simulink model "system_model"  (R2024b)
settings: Solver=VariableStepAuto  StartTime=0.0  StopTime=50  RelTol=1e-3
values from neighbouring files (symbols this model uses):
  a = -21212/c    (= -13.249219238)    [Controller.m]    (also in Controller2.m; Controller_motor_only.m = -15.4812967581; motor_control.m)
  b = 21104/c    (= 13.1817613991)    [Controller.m]    (also in Controller2.m; Controller_motor_only.m = 15.421446384; motor_control.m)
  d = -1599/c    (= -0.998750780762)    [Controller.m]    (also in Controller2.m; Controller_motor_only.m = 0.995012468828; motor_control.m)
  K = -F(1:2)    [State_Space_Controller.m]
  N = -F(3)    [State_Space_Controller.m]
  Ts = 0.01    [Controller.m]    (also in Controller2.m; Controller_motor_only.m; State_Space_Controller.m; dist_translate.m)
undefined symbols (not defined in the file or in its folder): dspblkCoreblockFVToolHelper, gcbh
libraries: cstblocks x2
settings Model: Creator=alexb  LastModifiedBy=ethan

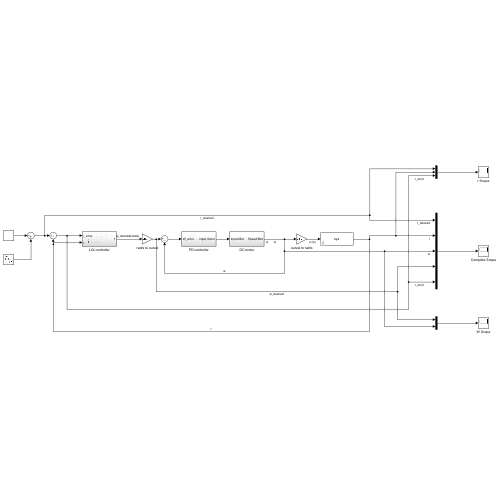
[thumbnail: Simulink's stored preview of the top-level diagram]
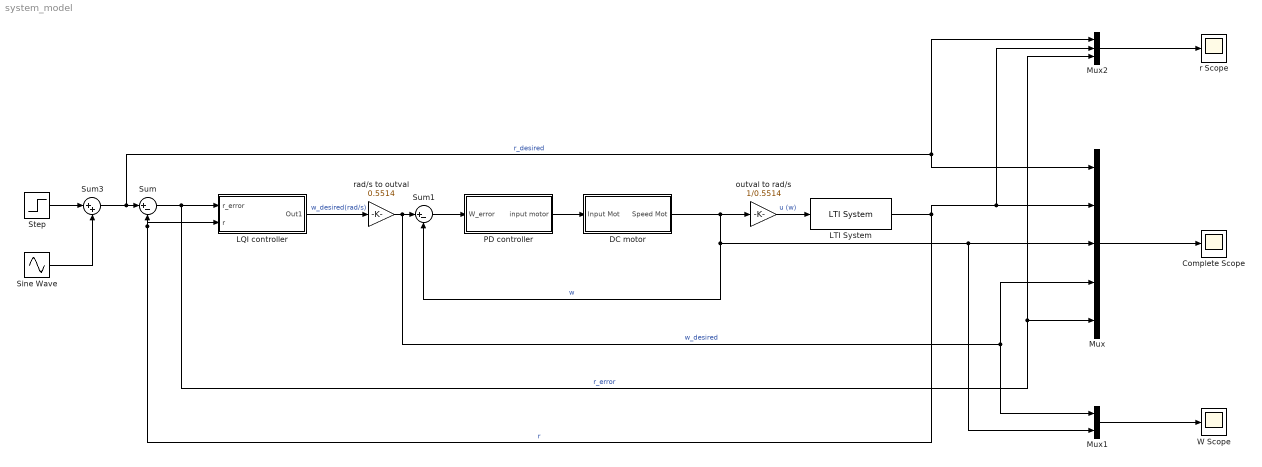
== system system_model ==
  Complete Scope : Scope
  DC motor : Subsystem
  LQI controller : Subsystem
  LTI System : cstblocks/LTI System  sys=sys  IC=[]  PadeOrder=0
  Mux : Mux  Inputs=5
  Mux1 : Mux  Inputs=2
  Mux2 : Mux  Inputs=3
  PD controller : Subsystem
  Sine Wave : Sin  Amplitude=0  Frequency=0.5  SampleTime=0
  Step : Step  Time=20  Before=0.1  After=0.13  SampleTime=0
  Sum : Sum  Inputs=|+-
  Sum1 : Sum  Inputs=|+-
  Sum3 : Sum  Inputs=|++
  W Scope : Scope
  outval to rad/s : Gain  Gain=1/0.5514
  r Scope : Scope
  rad/s to outval : Gain  Gain=0.5514
  wires:
  Sum1/1 -> PD controller/1(W_error)
  PD controller/1(input motor) -> DC motor/1(Input Mot)
  DC motor/1(Speed Mot) -> outval to rad/s/1, Mux/3, Mux1/2, Sum1/2  "w"
  Mux/1 -> Complete Scope/1
  Sum/1 -> Mux/5, Mux2/3, LQI controller/1(r_error)  "r_error"
  Step/1 -> Sum3/1
  LTI System/1 -> Mux2/2, Mux/2, Sum/2, LQI controller/2(r)  "r"
  LQI controller/1(Out1) -> rad/s to outval/1  "w_desired(rad/s)"
  Mux1/1 -> W Scope/1
  Mux2/1 -> r Scope/1
  Sum3/1 -> Mux/1, Mux2/1, Sum/1  "r_desired"
  Sine Wave/1 -> Sum3/2
  outval to rad/s/1 -> LTI System/1  "u (w)"
  rad/s to outval/1 -> Mux/4, Mux1/1, Sum1/1  "w_desired"

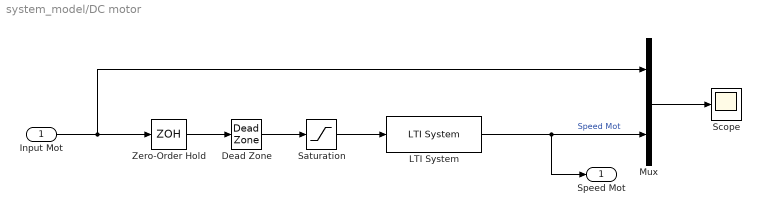
== system system_model/DC motor ==
  Input Mot : Inport
  Dead Zone : DeadZone  LowerValue=-1.75  UpperValue=1.7
  LTI System : cstblocks/LTI System  sys=Mc  IC=[]  PadeOrder=0
  Mux : Mux  Inputs=2
  Saturation : Saturate  UpperLimit=8.30  LowerLimit=-8.42
  Scope : Scope
  Zero-Order Hold : ZeroOrderHold  SampleTime=0.01
  Speed Mot : Outport
  wires:
  Input Mot/1 -> Mux/1, Zero-Order Hold/1
  Mux/1 -> Scope/1
  LTI System/1 -> Speed Mot/1, Mux/2  "Speed Mot"
  Dead Zone/1 -> Saturation/1
  Zero-Order Hold/1 -> Dead Zone/1
  Saturation/1 -> LTI System/1

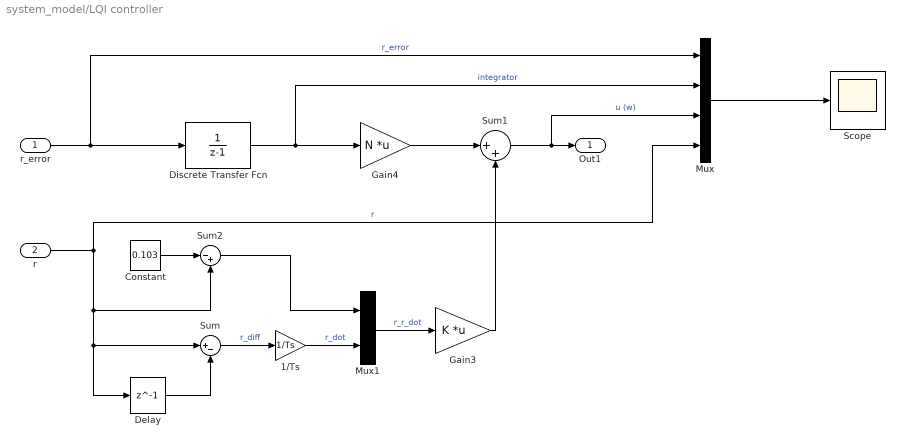
== system system_model/LQI controller ==
  r_error : Inport
  r : Inport  Port=2
  1/Ts : Gain  Gain=1/Ts
  Constant : Constant  Value=0.103
  Delay : Delay  DelayLength=1  InputProcessing=Columns as channels (frame based)
  Discrete Transfer Fcn : DiscreteTransferFcn  LoadFcn=dspblkCoreblockFVToolHelper(gcbh,'load');  Denominator=[1 -1]
      settings: CopyFcn=dspblkCoreblockFVToolHelper(gcbh,'copy');  DeleteFcn=dspblkCoreblockFVToolHelper(gcbh,'close');  ModelCloseFcn=dspblkCoreblockFVToolHelper(gcbh,'close');  PreSaveFcn=dspblkCoreblockFVToolHelper(gcbh,'presave');  PostSaveFcn=dspblkCoreblockFVToolHelper(gcbh,'postsave');  CloseFcn=dspblkCoreblockFVToolHelper(gcbh,'close');
  Gain3 : Gain  Gain=K  Multiplication=Matrix(K*u)
  Gain4 : Gain  Gain=N  Multiplication=Matrix(K*u)
  Mux : Mux
  Mux1 : Mux  Inputs=2
  Scope : Scope
  Sum : Sum  Inputs=|+-
  Sum1 : Sum  Inputs=|++
  Sum2 : Sum  Inputs=|-+
  Out1 : Outport
  wires:
  Mux/1 -> Scope/1
  Discrete Transfer Fcn/1 -> Mux/2, Gain4/1  "integrator"
  Gain3/1 -> Sum1/2
  Sum1/1 -> Out1/1, Mux/3  "u (w)"
  r_error/1 -> Discrete Transfer Fcn/1, Mux/1  "r_error"
  Gain4/1 -> Sum1/1
  r/1 -> Delay/1, Sum/1, Sum2/2, Mux/4  "r"
  Delay/1 -> Sum/2
  Mux1/1 -> Gain3/1  "r_r_dot"
  Sum/1 -> 1/Ts/1  "r_diff"
  1/Ts/1 -> Mux1/2  "r_dot"
  Sum2/1 -> Mux1/1
  Constant/1 -> Sum2/1

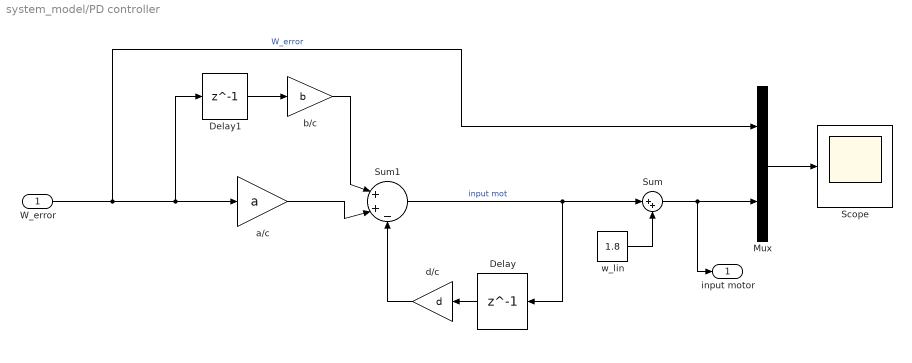
== system system_model/PD controller ==
  W_error : Inport
  Delay : Delay  DelayLength=1  InputProcessing=Columns as channels (frame based)
  Delay1 : Delay  DelayLength=1  InputProcessing=Columns as channels (frame based)
  Mux : Mux  Inputs=2
  Scope : Scope
  Sum : Sum  Inputs=|++
  Sum1 : Sum  Inputs=|++-
  a/c : Gain  Gain=a
  b/c : Gain  Gain=b
  d/c : Gain  Gain=d
  w_lin : Constant  Value=1.8
  input motor : Outport
  wires:
  Sum1/1 -> Sum/1, Delay/1  "input mot"
  b/c/1 -> Sum1/1
  d/c/1 -> Sum1/3
  Mux/1 -> Scope/1
  Delay/1 -> d/c/1
  a/c/1 -> Sum1/2
  W_error/1 -> a/c/1, Delay1/1, Mux/1  "W_error"
  Delay1/1 -> b/c/1
  Sum/1 -> input motor/1, Mux/2
  w_lin/1 -> Sum/2
